simulink model "jsbsimgui_test"  (Simulink 7.2)
settings: Solver=ode3  StartTime=0.0  StopTime=5  FixedStep=1/120  RelTol=1e-3
undefined symbols (not defined in the file or in its folder): init_aileron, init_elevator, init_flaps, init_gear, init_mixture, init_rudder, init_run_set, init_throttle
settings Model: Creator=Bri  LastModifiedBy=BRIAN
settings DataIOCC: SaveState=on

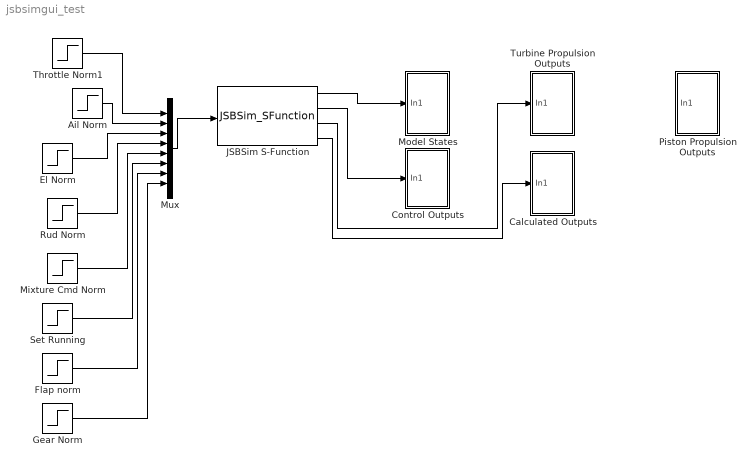
== system jsbsimgui_test ==
  Ail Norm : Step  Time=3  Before=init_aileron  After=init_aileron  SampleTime=0
  Calculated Outputs : Subsystem
  Control Outputs : Subsystem
  El Norm : Step  Time=15  Before=init_elevator  After=init_elevator  SampleTime=0
  Flap norm : Step  Time=0  Before=init_flaps  After=init_flaps  SampleTime=0
  Gear Norm : Step  Time=0  Before=init_gear  After=init_gear  SampleTime=0
  JSBSim S-Function : S-Function  FunctionName=JSBSim_SFunction  Parameters=ac_name, IC_states, IC_controls, IC_delta_t, IC_verbosity,IC_sim_multiplier  EnableBusSupport=off  mask{ac_name='t38', IC_states=[ 614.9985 0 0 0 0 0 20000 122 34 0 -0.06 0 ], IC_controls=[ 0.97915 0 0.02 0 0.7 1 0 0 ], IC_delta_t=0.00833, IC_verbosity='verbose', IC_sim_multiplier=1}
      mask prompts: ac_name "AC:"; IC_states "States:"; IC_controls "Controls:"; IC_delta_t "Delta:"; IC_verbosity "Verbosity:"; IC_sim_multiplier "JSBSim Multiplier:"
  Mixture Cmd Norm : Step  Time=.1  Before=init_mixture  After=init_mixture  SampleTime=0
  Model States : Subsystem
  Mux : Mux  Inputs=8
  Piston Propulsion Outputs : Subsystem
  Rud Norm : Step  Time=5  Before=init_rudder  After=init_rudder  SampleTime=0
  Set Running : Step  Time=0  Before=init_run_set  After=init_run_set  SampleTime=0
  Throttle Norm1 : Step  Time=0  Before=init_throttle  After=init_throttle  SampleTime=0
  Turbine Propulsion Outputs : Subsystem
  wires:
  Mux/1 -> JSBSim S-Function/1
  Throttle Norm1/1 -> Mux/1
  El Norm/1 -> Mux/3
  Rud Norm/1 -> Mux/4
  Mixture Cmd Norm/1 -> Mux/5
  Set Running/1 -> Mux/6
  Flap norm/1 -> Mux/7
  Gear Norm/1 -> Mux/8
  Ail Norm/1 -> Mux/2
  JSBSim S-Function/1 -> Model States/1(In1)
  JSBSim S-Function/2 -> Control Outputs/1(In1)
  JSBSim S-Function/3 -> Turbine Propulsion Outputs/1(In1)
  JSBSim S-Function/4 -> Calculated Outputs/1(In1)

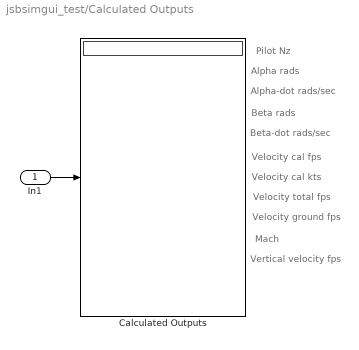
== system jsbsimgui_test/Calculated Outputs ==
  note: Pilot Nz
  note: Alpha rads
  note: Alpha-dot rads/sec
  note: Beta rads
  note: Beta-dot rads/sec
  note: Velocity cal fps
  note: Velocity cal kts
  note: Velocity total fps
  note: Velocity ground fps
  note: Mach
  note: Vertical velocity fps
  In1 : Inport
  Calculated Outputs : Display
  wires:
  In1/1 -> Calculated Outputs/1

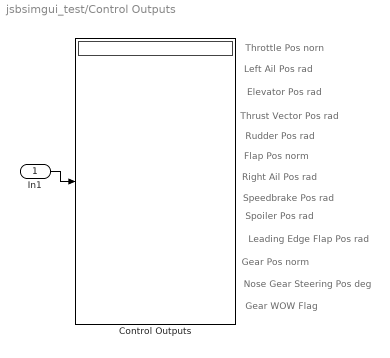
== system jsbsimgui_test/Control Outputs ==
  note: Throttle Pos norn
  note: Left Ail Pos rad
  note: Elevator Pos rad
  note: Rudder Pos rad
  note: Thrust Vector Pos rad
  note: Flap Pos norm
  note: Right Ail Pos rad
  note: Speedbrake Pos rad
  note: Spoiler Pos rad
  note: Leading Edge Flap Pos rad
  note: Gear Pos norm
  note: Nose Gear Steering Pos deg
  note: Gear WOW Flag
  In1 : Inport
  Control Outputs : Display
  wires:
  In1/1 -> Control Outputs/1

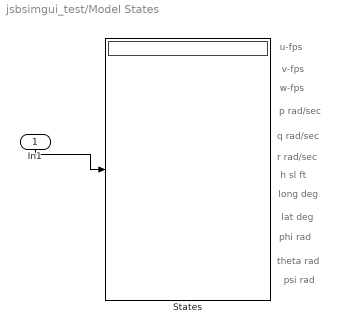
== system jsbsimgui_test/Model States ==
  note: u-fps
  note: v-fps
  note: w-fps
  note: p rad/sec
  note: q rad/sec
  note: r rad/sec
  note: h sl ft
  note: long deg
  note: lat deg
  note: phi rad
  note: theta rad
  note: psi rad
  In1 : Inport  Orientation=down
  States : Display
  wires:
  In1/1 -> States/1

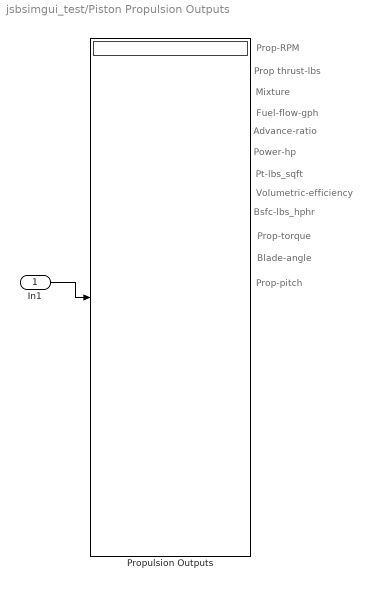
== system jsbsimgui_test/Piston Propulsion Outputs ==
  note: Prop-RPM
  note: Prop thrust-lbs
  note: Mixture
  note: Fuel-flow-gph
  note: Advance-ratio
  note: Power-hp
  note: Pt-lbs_sqft
  note: Bsfc-lbs_hphr
  note: Volumetric-efficiency
  note: Prop-torque
  note: Blade-angle
  note: Prop-pitch
  In1 : Inport
  Propulsion Outputs : Display
  wires:
  In1/1 -> Propulsion Outputs/1

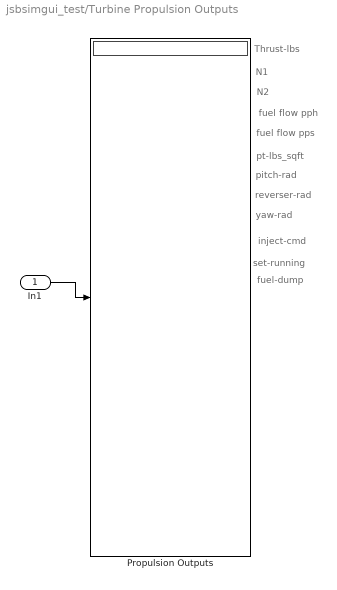
== system jsbsimgui_test/Turbine Propulsion Outputs ==
  note: Thrust-lbs
  note: N1
  note: N2
  note: fuel flow pph
  note: fuel flow pps
  note: pt-lbs_sqft
  note: pitch-rad
  note: reverser-rad
  note: yaw-rad
  note: inject-cmd
  note: set-running
  note: fuel-dump
  In1 : Inport
  Propulsion Outputs : Display
  wires:
  In1/1 -> Propulsion Outputs/1
